simulink model "fase1"  (Simulink 8.7)
settings: Solver=VariableStepAuto  StartTime=0.0  StopTime=60  RelTol=1e-3
values from neighbouring files (symbols this model uses):
  M = 70    [CG.m]    (also in odefun2.m = [w.Jr+(w.Mr+w.M)*(w.R^2)     w.M*w.R*w.l*cos(y(1)))
undefined symbols (not defined in the file or in its folder): F, Fr, Jr, R, Rl
libraries: fuzblock x1
settings Model: Creator=egualter  LastModifiedBy=egualter
settings DataIOCC: LimitDataPoints=off  SaveFormat=Dataset
settings DebuggingCC: UnderspecifiedInitializationDetection=Simplified  MergeDetectMultiDrivingBlocksExec=error
settings HardwareCC: ProdBitPerPointer=64  ProdLargestAtomicFloat=Float  ProdIntDivRoundTo=Zero  ProdEndianess=LittleEndian  ProdWordSize=64  ProdHWDeviceType=Intel->x86-64 (Windows64)
settings ModelReferenceCC: PropagateSignalLabelsOutOfModel=on
settings ConfigComp: CovModelRefEnable=off

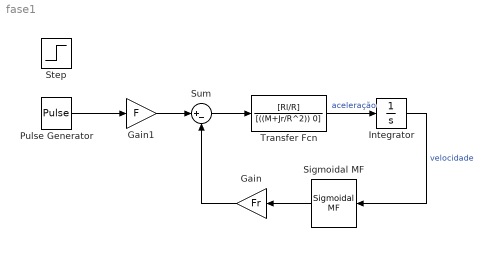
== system fase1 ==
  Gain : Gain  Gain=Fr
  Gain1 : Gain  Gain=F
  Integrator : Integrator
  Pulse Generator : DiscretePulseGenerator  PulseType=Time based  Period=25  PulseWidth=10
  Sigmoidal MF : fuzblock/Membership  Functions/Sigmoidal MF  a=0.5  c=1
  Step : Step  SampleTime=0
  Sum : Sum  Inputs=|+-
  Transfer Fcn : TransferFcn  Numerator=[Rl/R]  Denominator=[((M+Jr/R^2)) 0]
  wires:
  Sum/1 -> Transfer Fcn/1
  Transfer Fcn/1 -> Integrator/1  "aceleração"
  Integrator/1 -> Sigmoidal MF/1  "velocidade"
  Gain/1 -> Sum/2
  Gain1/1 -> Sum/1
  Sigmoidal MF/1 -> Gain/1
  Pulse Generator/1 -> Gain1/1
